simulink model "sim_ex2"  (R2015b)
settings: Solver=ode23t  StartTime=0.0  StopTime=simtime  RelTol=1e-3
values from neighbouring files (symbols this model uses):
  enable_sin = 1    [ex1.m]    (also in ex2.m = 0; ex3.m; ex4.m = 0; exall.m = 0)
  J = (J1 + J2)    (= 3.6e-05)    [ex1.m]    (also in ex2.m; ex3.m; ex4.m)
  motor_L = motor_pars    [ex1.m]    (also in ex2.m; ex3.m; ex4.m)
  n = 5    [ex1.m]    (also in ex2.m; ex3.m; ex4.m; ex5.m)
  sim_step_v = 2.38    [ex1.m]    (also in ex2.m = 1; ex3.m; ex4.m = 10)
undefined symbols (not defined in the file or in its folder): T_fric
settings Model: Creator=gabras  LastModifiedBy=Andreas
settings SolverCC: ZeroCrossAlgorithm=Adaptive
settings DataIOCC: SaveFormat=Array
settings DebuggingCC: SolverPrmCheckMsg=warning
settings HardwareCC: ProdBitPerPointer=32  ProdLargestAtomicFloat=None  ProdIntDivRoundTo=Undefined  ProdEndianess=Unspecified  ProdWordSize=32  ProdHWDeviceType=32-bit Generic
settings GRTTargetCC: GeneratePreprocessorConditionals=Disable all
settings ConfigComp: CovModelRefEnable=Off  CovSFcnEnable=off

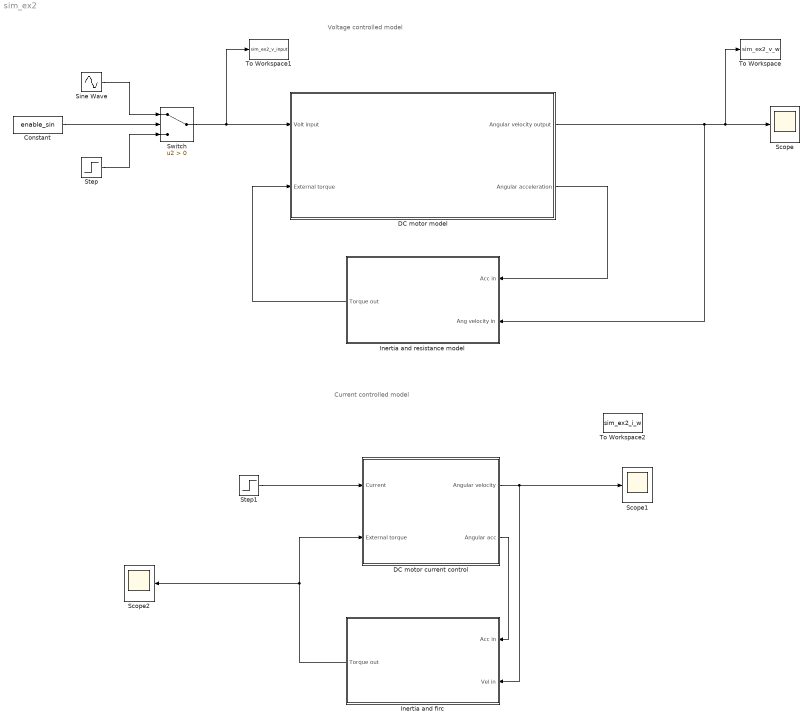
== system sim_ex2 ==
  note: Current controlled model
  note: Voltage controlled model
  Constant : Constant  Value=enable_sin
  "DC motor current control " : Subsystem
  DC motor model : Subsystem
  Inertia and firc : Subsystem
  "Inertia and resistance model " : Subsystem
  Scope : Scope
  Scope1 : Scope
  Scope2 : Scope
  Sine Wave : Sin  SampleTime=0
  Step : Step  Time=0  After=sim_step_v  SampleTime=0
  Step1 : Step  Time=0  SampleTime=0
  Switch : Switch  Criteria=u2 > Threshold
  To Workspace : ToWorkspace  VariableName=sim_ex2_v_w  SaveFormat=Timeseries  SampleTime=-1
  To Workspace1 : ToWorkspace  VariableName=sim_ex2_v_input  SaveFormat=Timeseries  SampleTime=-1
  To Workspace2 : ToWorkspace  VariableName=sim_ex2_i_w  SaveFormat=Timeseries  SampleTime=-1
  wires:
  DC motor model/1("Angular velocity output ") -> "Inertia and resistance model "/2(Ang velocity in), To Workspace/1, Scope/1
  "Inertia and resistance model "/1(Torque out) -> DC motor model/2(External torque)
  DC motor model/2("Angular acceleration ") -> "Inertia and resistance model "/1(Acc in)
  Step1/1 -> "DC motor current control "/1(Current)
  "DC motor current control "/1(Angular velocity) -> Scope1/1, Inertia and firc/2(Vel in)
  "DC motor current control "/2(Angular acc) -> Inertia and firc/1(Acc in)
  Inertia and firc/1(Torque out) -> Scope2/1, "DC motor current control "/2(External torque)
  Step/1 -> Switch/3
  Sine Wave/1 -> Switch/1
  Switch/1 -> To Workspace1/1, DC motor model/1("Volt input ")
  Constant/1 -> Switch/2

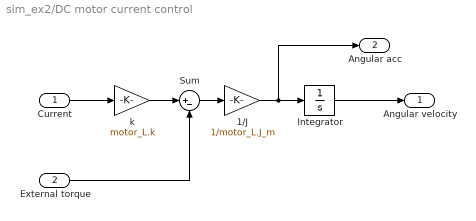
== system sim_ex2/DC motor current control  ==
  Current : Inport
  External torque : Inport  Port=2
  1/J : Gain  Gain=1/motor_L.J_m
  Integrator : Integrator
  Sum : Sum  Inputs=|+-
  "k " : Gain  Gain=motor_L.k
  Angular velocity : Outport
  Angular acc : Outport  Port=2
  wires:
  Current/1 -> "k "/1
  External torque/1 -> Sum/2
  "k "/1 -> Sum/1
  Sum/1 -> 1/J/1
  1/J/1 -> Angular acc/1, Integrator/1
  Integrator/1 -> Angular velocity/1

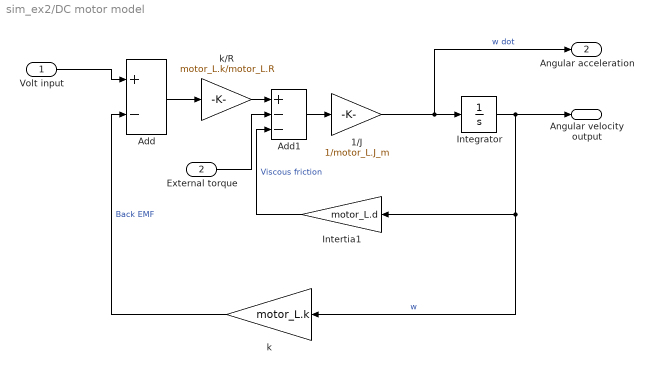
== system sim_ex2/DC motor model ==
  "Volt input " : Inport
  External torque : Inport  Port=2
  1/J : Gain  Gain=1/motor_L.J_m
  Add : Sum  Inputs=+-
  Add1 : Sum  Inputs=+--
  Integrator : Integrator
  Intertia1 : Gain  Gain=motor_L.d
  k : Gain  Gain=motor_L.k
  "k/R " : Gain  Gain=motor_L.k/motor_L.R
  "Angular velocity output " : Outport
  "Angular acceleration " : Outport  Port=2
  wires:
  "Volt input "/1 -> Add/1
  k/1 -> Add/2  "Back EMF"
  Add/1 -> "k/R "/1
  "k/R "/1 -> Add1/1
  Add1/1 -> 1/J/1
  1/J/1 -> "Angular acceleration "/1, Integrator/1  "w dot"
  Integrator/1 -> "Angular velocity output "/1, k/1, Intertia1/1  "w"
  External torque/1 -> Add1/2
  Intertia1/1 -> Add1/3  "Viscous friction"

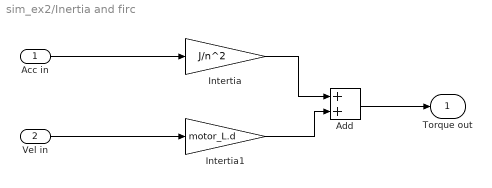
== system sim_ex2/Inertia and firc ==
  Acc in : Inport
  Vel in : Inport  Port=2
  Add : Sum
  Intertia : Gain  Gain=J/n^2
  Intertia1 : Gain  Gain=motor_L.d
  Torque out : Outport
  wires:
  Acc in/1 -> Intertia/1
  Vel in/1 -> Intertia1/1
  Intertia/1 -> Add/1
  Intertia1/1 -> Add/2
  Add/1 -> Torque out/1

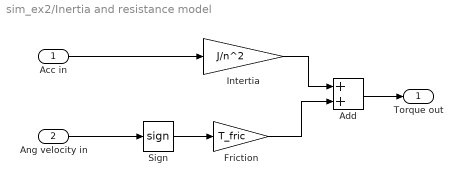
== system sim_ex2/Inertia and resistance model  ==
  Acc in : Inport
  Ang velocity in : Inport  Port=2
  Add : Sum
  Friction : Gain  Gain=T_fric
  Intertia : Gain  Gain=J/n^2
  Sign : Signum
  Torque out : Outport
  wires:
  Acc in/1 -> Intertia/1
  Ang velocity in/1 -> Sign/1
  Sign/1 -> Friction/1
  Add/1 -> Torque out/1
  Intertia/1 -> Add/1
  Friction/1 -> Add/2
